simulink model "DaVinci_CLIK"  (R2023a)
settings: Solver=VariableStepAuto  StartTime=0.0  StopTime=10.0  RelTol=1e-3
undefined symbols (not defined in the file): q
libraries: DaVinci_Lib x2, DaVinci_LibJ x1
settings Model: Creator=afons  LastModifiedBy=afons

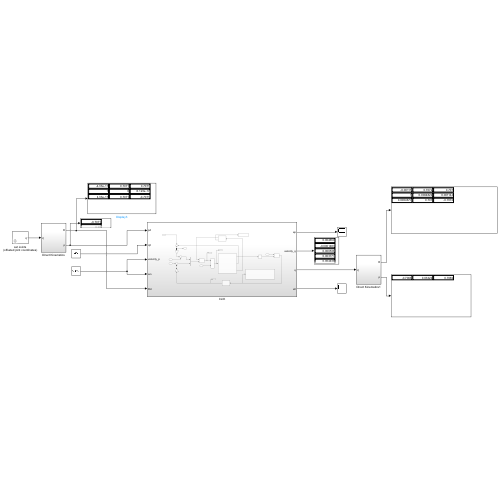
[thumbnail: Simulink's stored preview of the top-level diagram]
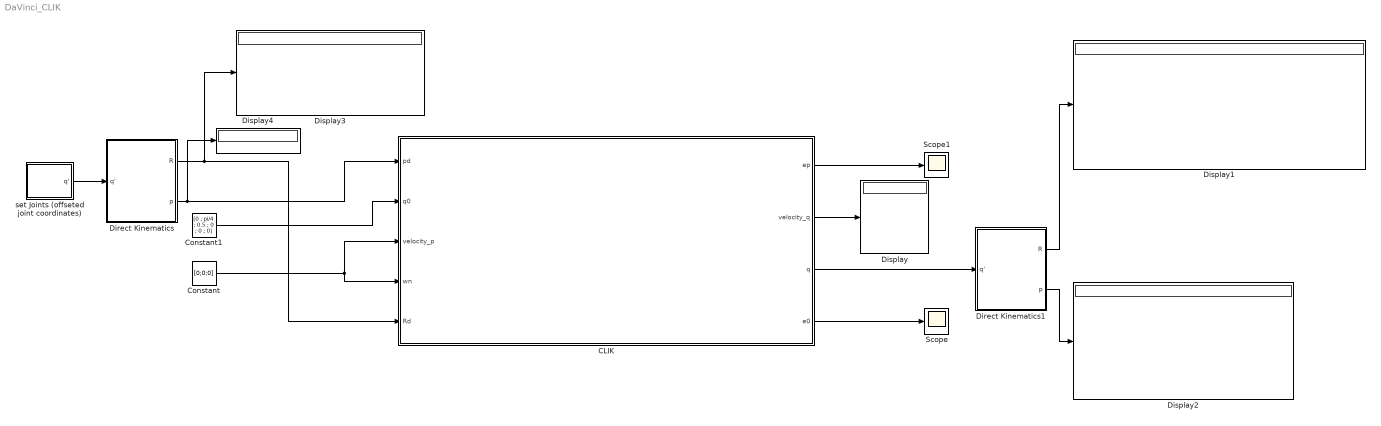
== system DaVinci_CLIK ==
  CLIK : Subsystem
  Constant : Constant  Value=[0;0;0]
  Constant1 : Constant  Value=[0 ; pi/4 ; 0.5 ; 0 ; 0 ; 0]
  Direct Kinematics : Subsystem
  Direct Kinematics1 : Subsystem
  Display{,1..4} (5 alike) : Display
  Scope : Scope
  Scope1 : Scope
  set Joints (offseted joint coordinates) : Subsystem  mask{q1=0, q2=45, q3=1, q4=0, q5=90, q6=0}
  wires:
  Direct Kinematics/1(R) -> Display3/1, CLIK/5(Rd)
  Direct Kinematics/2(p) -> Display4/1, CLIK/1(pd)
  Constant/1 -> CLIK/3(velocity_p), CLIK/4(wn)
  Constant1/1 -> CLIK/2(q0)
  CLIK/4(e0) -> Scope/1
  CLIK/1(ep) -> Scope1/1
  set Joints (offseted joint coordinates)/1(q') -> Direct Kinematics/1(q')
  CLIK/3(q) -> Direct Kinematics1/1(q')
  CLIK/2(velocity_q) -> Display/1
  Direct Kinematics1/2(p) -> Display2/1
  Direct Kinematics1/1(R) -> Display1/1

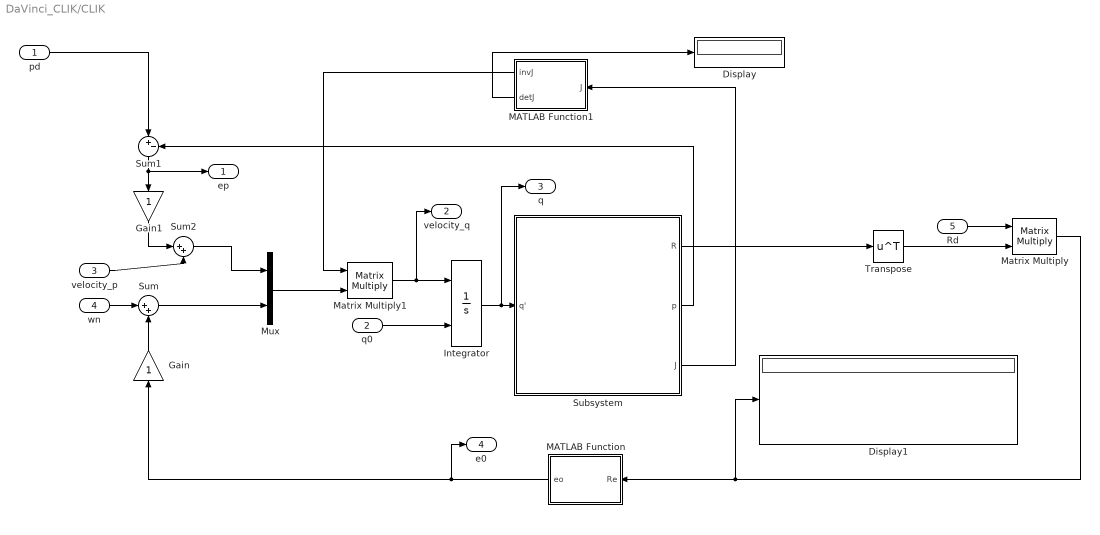
== system DaVinci_CLIK/CLIK ==
  pd : Inport
  q0 : Inport  Port=2
  velocity_p : Inport  Port=3
  wn : Inport  Port=4
  Rd : Inport  Port=5
  Display : Display
  Display1 : Display
  Gain : Gain
  Gain1 : Gain
  Integrator : Integrator  InitialConditionSource=external  InitialCondition=q(0)
  MATLAB Function : MATLAB Function  TreatAsAtomicUnit=on
  MATLAB Function1 : MATLAB Function  TreatAsAtomicUnit=on
  Matrix Multiply : Product  Multiplication=Matrix(*)
  Matrix Multiply1 : Product  Multiplication=Matrix(*)
  Mux : Mux  Inputs=2
  Subsystem : Subsystem
  Sum : Sum  Inputs=|++
  Sum1 : Sum  Inputs=|+-
  Sum2 : Sum  Inputs=|++
  Transpose : Math  Operator=transpose
  ep : Outport
  velocity_q : Outport  Port=2
  q : Outport  Port=3
  e0 : Outport  Port=4
  wires:
  Matrix Multiply/1 -> Display1/1, MATLAB Function/1(Re)
  Gain1/1 -> Sum2/1
  Subsystem/1(R) -> Transpose/1
  Sum1/1 -> ep/1, Gain1/1
  Gain/1 -> Sum/2
  MATLAB Function/1(eo) -> e0/1, Gain/1
  MATLAB Function1/2(detJ) -> Display/1
  Sum2/1 -> Mux/1
  Sum/1 -> Mux/2
  Subsystem/3(J) -> MATLAB Function1/1(J)
  Subsystem/2(p) -> Sum1/2
  Integrator/1 -> q/1, Subsystem/1(q')
  Matrix Multiply1/1 -> velocity_q/1, Integrator/1
  Transpose/1 -> Matrix Multiply/2
  MATLAB Function1/1(invJ) -> Matrix Multiply1/1
  Mux/1 -> Matrix Multiply1/2
  pd/1 -> Sum1/1
  Rd/1 -> Matrix Multiply/1
  wn/1 -> Sum/1
  velocity_p/1 -> Sum2/2
  q0/1 -> Integrator/2

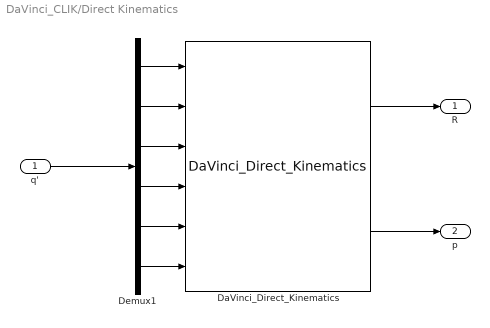
== system DaVinci_CLIK/Direct Kinematics ==
  q' : Inport
  DaVinci_Direct_Kinematics : DaVinci_Lib/DaVinci_Direct_Kinematics  SystemSampleTime=-1  VariantActivationTime=update diagram  Latency=0  AutoFrameSizeCalculation=off
  Demux1 : Demux  Outputs=6
  R : Outport
  p : Outport  Port=2
  wires:
  DaVinci_Direct_Kinematics/1 -> R/1
  DaVinci_Direct_Kinematics/2 -> p/1
  q'/1 -> Demux1/1
  Demux1/6 -> DaVinci_Direct_Kinematics/6
  Demux1/1 -> DaVinci_Direct_Kinematics/1
  Demux1/4 -> DaVinci_Direct_Kinematics/4
  Demux1/2 -> DaVinci_Direct_Kinematics/2
  Demux1/5 -> DaVinci_Direct_Kinematics/5
  Demux1/3 -> DaVinci_Direct_Kinematics/3

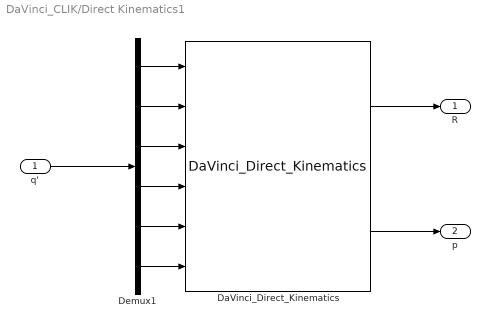
== system DaVinci_CLIK/Direct Kinematics1 ==
  q' : Inport
  DaVinci_Direct_Kinematics : DaVinci_Lib/DaVinci_Direct_Kinematics  SystemSampleTime=-1  VariantActivationTime=update diagram  Latency=0  AutoFrameSizeCalculation=off
  Demux1 : Demux  Outputs=6
  R : Outport
  p : Outport  Port=2
  wires:
  DaVinci_Direct_Kinematics/1 -> R/1
  DaVinci_Direct_Kinematics/2 -> p/1
  q'/1 -> Demux1/1
  Demux1/6 -> DaVinci_Direct_Kinematics/6
  Demux1/1 -> DaVinci_Direct_Kinematics/1
  Demux1/4 -> DaVinci_Direct_Kinematics/4
  Demux1/2 -> DaVinci_Direct_Kinematics/2
  Demux1/5 -> DaVinci_Direct_Kinematics/5
  Demux1/3 -> DaVinci_Direct_Kinematics/3

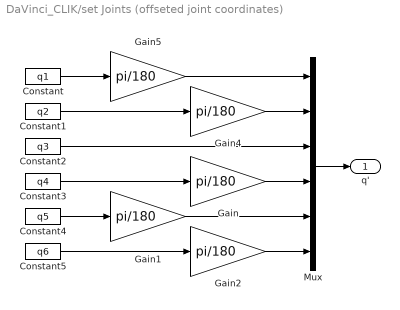
== system DaVinci_CLIK/set Joints (offseted joint coordinates) ==
  Constant : Constant  Value=q1
  Constant1 : Constant  Value=q2
  Constant2 : Constant  Value=q3
  Constant3 : Constant  Value=q4
  Constant4 : Constant  Value=q5
  Constant5 : Constant  Value=q6
  Gain{,1..2,4..5} (5 alike) : Gain  Gain=pi/180
  Mux : Mux  Inputs=6
  q' : Outport
  wires:
  Gain2/1 -> Mux/6
  Constant1/1 -> Gain4/1
  Constant3/1 -> Gain/1
  Constant5/1 -> Gain2/1
  Mux/1 -> q'/1
  Gain5/1 -> Mux/1
  Gain/1 -> Mux/4
  Gain1/1 -> Mux/5
  Gain4/1 -> Mux/2
  Constant/1 -> Gain5/1
  Constant2/1 -> Mux/3
  Constant4/1 -> Gain1/1

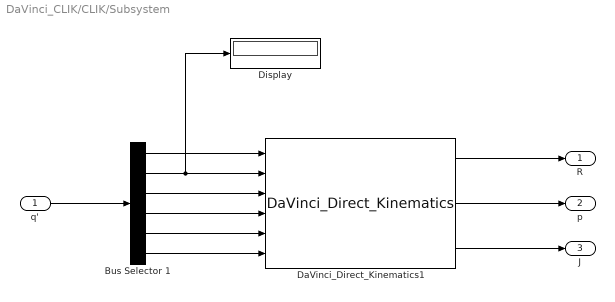
== system DaVinci_CLIK/CLIK/Subsystem ==
  q' : Inport
  Bus Selector 1 : Demux  Outputs=6
  DaVinci_Direct_Kinematics1 : DaVinci_LibJ/DaVinci_Direct_Kinematics  SystemSampleTime=-1  VariantActivationTime=update diagram  Latency=0  AutoFrameSizeCalculation=off
      settings: LibrarySourceBlock=|
      | simulink/User-Defined
      | Functions/MATLAB Function
  Display : Display
  R : Outport
  p : Outport  Port=2
  J : Outport  Port=3
  wires:
  Bus Selector 1/2 -> Display/1, DaVinci_Direct_Kinematics1/2
  Bus Selector 1/6 -> DaVinci_Direct_Kinematics1/6
  Bus Selector 1/3 -> DaVinci_Direct_Kinematics1/3
  Bus Selector 1/1 -> DaVinci_Direct_Kinematics1/1
  Bus Selector 1/5 -> DaVinci_Direct_Kinematics1/5
  Bus Selector 1/4 -> DaVinci_Direct_Kinematics1/4
  DaVinci_Direct_Kinematics1/1 -> R/1
  q'/1 -> Bus Selector 1/1
  DaVinci_Direct_Kinematics1/2 -> p/1
  DaVinci_Direct_Kinematics1/3 -> J/1

== matlab function DaVinci_CLIK/CLIK/MATLAB Function1 ==
  data: J input; invJ output; detJ output
function [invJ,detJ]  = invert(J)

detJ = det(J);
if -0.1 < detJ < 0.1
    invJ = J';
else
    invJ=inv(J);
end
end

== matlab function DaVinci_CLIK/CLIK/MATLAB Function ==
  data: Re input; eo output
function eo = orint_error(Re)

d=diag (Re);
idx=find(d == max(d));
i=idx (1);
id=eye (3,3);
tr=trace(Re);

if -1 < tr && tr < 3
    theta = acos ((trace(Re)-1)/2);
    r=[Re(3,2) - Re(2, 3) ;
        Re(1,3) - Re(3, 1);
        Re(2,1) - Re(1,2)]* (1/(2*sin(theta)));

elseif tr == -1
    theta=pi;
    r=(id(:,i)+Re(:,i))/sqrt (2+2*Re(i,i));
    
else
    theta=0; 
    r= [0 0 1]';
end
r=r./norm(r);
eo=theta*r;
end
